simulink model "moore_basic_chart"  (R2024a)
settings: Solver=ode45  StartTime=0.0  StopTime=inf  RelTol=1e-3  EnableMultiTasking=on
settings Model: Creator=nunkesser  LastModifiedBy=nunkesser
settings SolverCC: AlgebraicLoopSolver=TrustRegion
settings DataIOCC: LimitDataPoints=on  SaveFormat=Array  ReturnWorkspaceOutputs=off
settings OptimizationCC: LifeSpan=inf
settings DebuggingCC: SolverPrmCheckMsg=warning  UnconnectedInputMsg=warning  UnconnectedOutputMsg=warning  UnconnectedLineMsg=warning  SFUnexpectedBacktrackingDiag=warning  SFNoUnconditionalDefaultTransitionDiag=warning  SFExecutionAtInitializationDiag=none  ArithmeticOperatorsInVariantConditions=warning
settings HardwareCC: ProdBitPerPointer=32  ProdBitPerSizeT=32  ProdBitPerPtrDiffT=32  ProdLargestAtomicFloat=None  ProdIntDivRoundTo=Undefined  ProdEndianess=Unspecified  ProdWordSize=32  ProdHWDeviceType=32-bit Generic
settings ModelReferenceCC: PropagateSignalLabelsOutOfModel=off
settings SFSimCC: SimUseLocalCustomCode=off  CustomCodeUndefinedFunction=UseInterfaceOnly
settings RTWCC: RTWUseLocalCustomCode=off  GPUComputeCapability=3.5
settings CodeAppCC: StateflowObjectComments=on
settings GRTTargetCC: TargetLangStandard=C89/C90 (ANSI)
settings ConfigComp: CovMetricSettings=dw  CovSaveCumulativeToWorkspaceVar=on  CovSaveSingleToWorkspaceVar=on  CovExternalEMLEnable=off  CovSFcnEnable=off

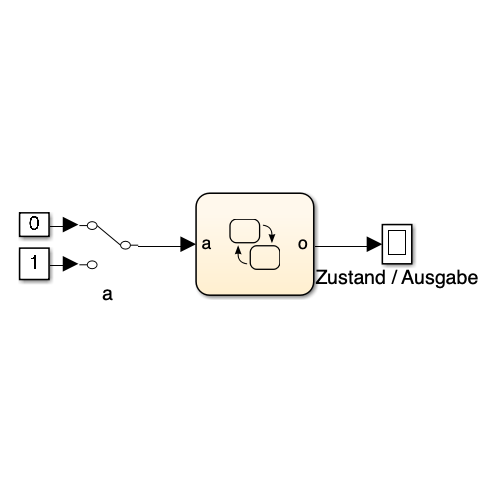
[thumbnail: Simulink's stored preview of the top-level diagram]
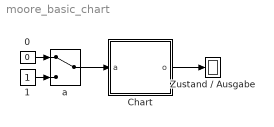
== system moore_basic_chart ==
  "0 " : Constant  Value=0  OutDataTypeStr=boolean
  1 : Constant  OutDataTypeStr=boolean
  Chart : Stateflow chart  TreatAsAtomicUnit=on
  Zustand / Ausgabe : Display
  a : ManualSwitch
  wires:
  1/1 -> a/2
  "0 "/1 -> a/1
  a/1 -> Chart/1(a)
  Chart/1(o) -> Zustand / Ausgabe/1

== stateflow chart moore_basic_chart/Chart ==
  state S0
    entry: o=0
  state S1
    entry: o=1
  (default) -> S0
  S1 -> S1 [order 2] : [a==0]
  S0 -> S1 [order 2] : [a==1]
  S0 -> S0 [order 1] : [a==0]
  S1 -> S0 [order 1] : [a==1]
  data: a input; o output
